simulink model "New_MPCI_JointSpace"  (R2023b)
settings: Solver=ode8  StartTime=0.0  StopTime=2  FixedStep=0.001  MaxStep=0.001  RelTol=1e-3
StopFcn:
  | clc
  | close all
  | plot(out.x_mpc,out.y_mpc,'LineWidth',1.5,'LineStyle','-.','Color','R')
  | hold on
  | plot(out.x_pid,out.y_pid,'LineWidth',1.5,'Color','B')
  | plot(out.x_d,out.y_d,'LineWidth',1.5,'LineStyle','--','Color','k')
  | legend('MPC','PID','Desired','Interpreter','tex','FontSize',15)
  | ax = gca;
  | xticklabels([-1.5 -1 -0.5 0 0.5 1 1.5 2 2.5])
  | yticklabels([141 141.5 142 142.5 143 143.5 144])
  | ax.XAxis.FontSize = 14;
  | ax.XAxis.FontWeight = 'bold';
  | ax = gca;
  | ax.YAxis.FontSize = 14;
  | ax.YAxis.FontWeight = 'bold';
  | xlabel('x(mm)','Interpreter','tex','FontSize',18,'FontWeight','bold');
  | ylabel('y(mm)','Interpreter','tex','FontSize',18,'FontWeight','bold');
  | title('End Effector Position','Interpreter','tex','FontSize',25,'FontWeight','bold');
  | grid on
  | hold off
libraries: slpidlib x1
(part 1 of 2)
settings Model: Creator=sinar  LastModifiedBy=sinar
settings SolverCC: InitialStep=0.001  ZeroCrossControl=DisableAll
settings DebuggingCC: UnconnectedInputMsg=warning  UnconnectedOutputMsg=warning  UnconnectedLineMsg=warning
settings ModelReferenceCC: EnableRefExpFcnMdlSchedulingChecks=on  ModelReferenceMinAlgLoopOccurrences=on
settings RTWCC: DLArmComputeVersion=19.05

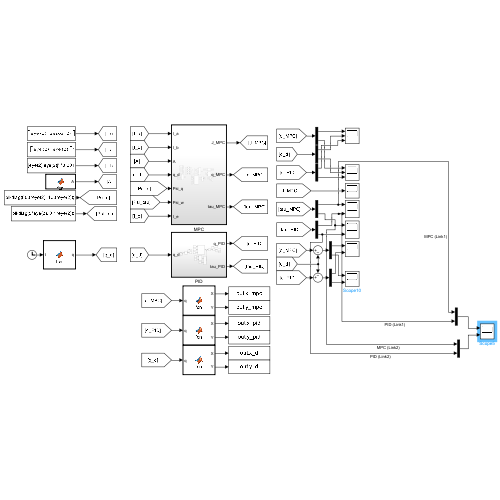
[thumbnail: Simulink's stored preview of the top-level diagram]
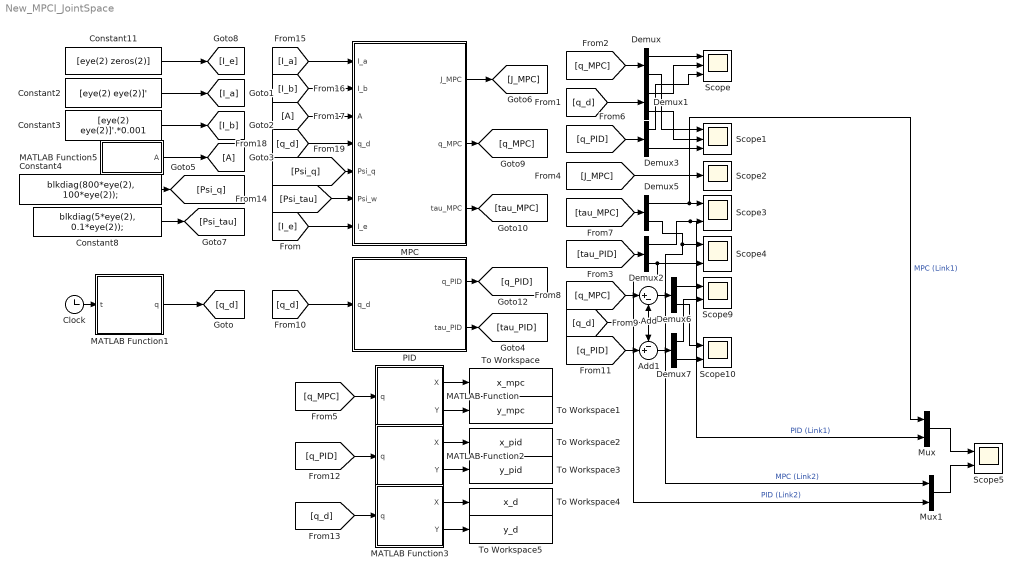
== system New_MPCI_JointSpace ==
  Add : Sum  Inputs=|+-
  Add1 : Sum  Inputs=-+|
  Clock : Clock
  Constant11 : Constant  Value=[eye(2) zeros(2)]
  Constant2 : Constant  Value=[eye(2) eye(2)]'
  Constant3 : Constant  Value=[eye(2) eye(2)]'.*0.001
  Constant4 : Constant  Value=blkdiag(800*eye(2), 100*eye(2));
  Constant8 : Constant  Value=blkdiag(5*eye(2), 0.1*eye(2));
  Demux{,1..3,5..7} (7 alike) : Demux  Outputs=2
  From17 : From
  Goto3 : Goto
  MATLAB Function : MATLAB Function  TreatAsAtomicUnit=on
  MATLAB Function1 : MATLAB Function  TreatAsAtomicUnit=on
  MATLAB Function2 : MATLAB Function  TreatAsAtomicUnit=on
  MATLAB Function3 : MATLAB Function  TreatAsAtomicUnit=on
  MATLAB Function5 : MATLAB Function  TreatAsAtomicUnit=on
  MPC : Subsystem  TreatAsAtomicUnit=on
      settings: MinAlgLoopOccurrences=on
  Mux : Mux  Inputs=2
  Mux1 : Mux  Inputs=2
  PID : Subsystem  TreatAsAtomicUnit=on
      settings: MinAlgLoopOccurrences=on
  Scope : Scope  NumInputPorts=3
  Scope1 : Scope  NumInputPorts=3
  Scope{3..5,9..10} (5 alike) : Scope  NumInputPorts=2
  Scope2 : Scope
  To Workspace : ToWorkspace  VariableName=x_mpc  SampleTime=-1
      settings: Save2DSignal=2-D array (concatenate along first dimension)
  To Workspace1 : ToWorkspace  VariableName=y_mpc  SampleTime=-1
      settings: Save2DSignal=2-D array (concatenate along first dimension)
  To Workspace2 : ToWorkspace  VariableName=x_pid  SampleTime=-1
      settings: Save2DSignal=2-D array (concatenate along first dimension)
  To Workspace3 : ToWorkspace  VariableName=y_pid  SampleTime=-1
      settings: Save2DSignal=2-D array (concatenate along first dimension)
  To Workspace4 : ToWorkspace  VariableName=x_d  SampleTime=-1
      settings: Save2DSignal=2-D array (concatenate along first dimension)
  To Workspace5 : ToWorkspace  VariableName=y_d  SampleTime=-1
      settings: Save2DSignal=2-D array (concatenate along first dimension)
  wires:
  MATLAB Function1/1(q) -> [q_d]
  Constant2/1 -> [I_a]
  Constant3/1 -> [I_b]
  MATLAB Function5/1(A) -> Goto3/1
  Constant4/1 -> [Psi_q]
  Constant8/1 -> [Psi_tau]
  Constant11/1 -> [I_e]
  MPC/1(J_MPC) -> [J_MPC]
  MPC/2(q_MPC) -> [q_MPC]
  MPC/3(tau_MPC) -> [tau_MPC]
  [Psi_tau] -> MPC/6(Psi_w)
  [Psi_q] -> MPC/5(Psi_q)
  [q_d] -> MPC/4(q_d)
  From17/1 -> MPC/3(A)
  [I_b] -> MPC/2(I_b)
  [I_a] -> MPC/1(I_a)
  Clock/1 -> MATLAB Function1/1(t)
  [I_e] -> MPC/7(I_e)
  Demux/1 -> Scope/1
  [q_d] -> Demux1/1
  [q_MPC] -> Demux/1
  [J_MPC] -> Scope2/1
  [tau_PID] -> Demux2/1
  [q_d] -> PID/1(q_d)
  PID/1(q_PID) -> [q_PID]
  PID/2(tau_PID) -> [tau_PID]
  [q_PID] -> Demux3/1
  [q_MPC] -> Add/1
  [q_d] -> Add/2, Add1/1
  [q_PID] -> Add1/2
  Add/1 -> Demux6/1
  Add1/1 -> Demux7/1
  Demux6/1 -> Scope9/1
  Demux7/1 -> Scope9/2
  Demux7/2 -> Scope10/2
  Demux6/2 -> Scope10/1
  [tau_MPC] -> Demux5/1
  Demux1/1 -> Scope/2
  Demux3/1 -> Scope/3
  Demux3/2 -> Scope1/3
  Demux1/2 -> Scope1/2
  Demux/2 -> Scope1/1
  MATLAB Function/1(X) -> To Workspace/1
  MATLAB Function/2(Y) -> To Workspace1/1
  [q_MPC] -> MATLAB Function/1(q)
  [q_PID] -> MATLAB Function2/1(q)
  MATLAB Function2/2(Y) -> To Workspace3/1
  MATLAB Function2/1(X) -> To Workspace2/1
  MATLAB Function3/1(X) -> To Workspace4/1
  MATLAB Function3/2(Y) -> To Workspace5/1
  [q_d] -> MATLAB Function3/1(q)
  Mux/1 -> Scope5/1
  Mux1/1 -> Scope5/2
  Demux2/2 -> Scope4/2, Mux1/2  "PID (Link2)"
  Demux5/2 -> Mux1/1, Scope4/1  "MPC (Link2)"
  Demux5/1 -> Mux/1, Scope3/1  "MPC (Link1)"
  Demux2/1 -> Mux/2, Scope3/2  "PID (Link1)"

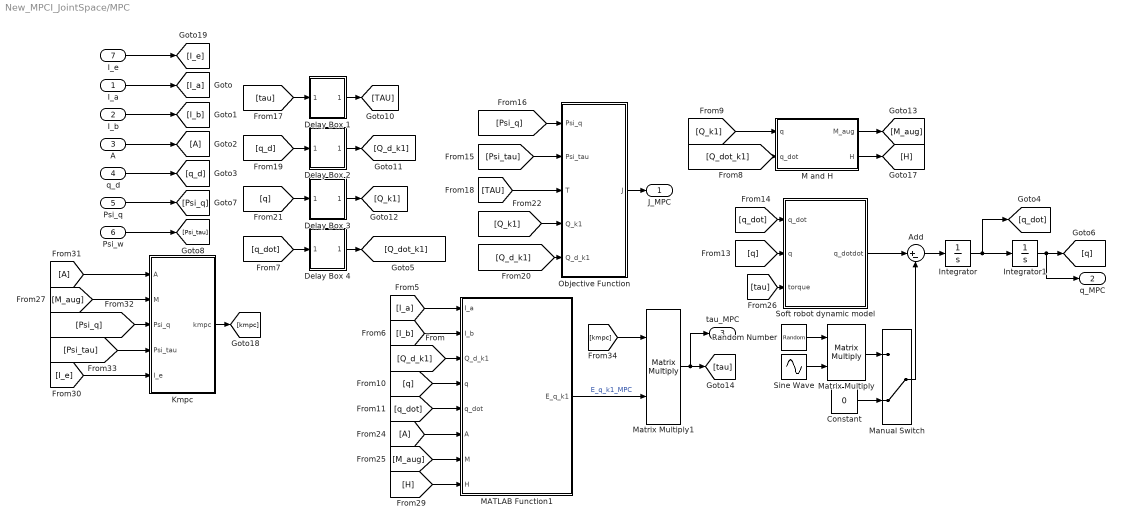
== system New_MPCI_JointSpace/MPC ==
  I_a : Inport
  I_b : Inport  Port=2
  A : Inport  Port=3
  q_d : Inport  Port=4
  Psi_q : Inport  Port=5
  Psi_w : Inport  Port=6
  I_e : Inport  Port=7
  Add : Sum  Inputs=|+-
  Constant : Constant  Value=0
  Delay Box 1 : Subsystem
  Delay Box 2 : Subsystem
  Delay Box 3 : Subsystem
  Delay Box 4 : Subsystem
  From24 : From
  From31 : From
  Goto2 : Goto
  Integrator : Integrator  InitialCondition=zeros(2,1)
  Integrator1 : Integrator  InitialCondition=[0.1 0.1]'
  Kmpc : MATLAB Function  TreatAsAtomicUnit=on
  M and H : MATLAB Function  TreatAsAtomicUnit=on
  MATLAB Function1 : MATLAB Function  TreatAsAtomicUnit=on
  Manual Switch : ManualSwitch  CurrentSetting=0
  Matrix Multiply : Product  Multiplication=Matrix(*)
  Matrix Multiply1 : Product  Multiplication=Matrix(*)
  Objective Function : MATLAB Function  TreatAsAtomicUnit=on
  Random Number : RandomNumber  Variance=5  SampleTime=0.01
  Sine Wave : Sin  Amplitude=10  Frequency=10  SampleTime=0
  Soft robot dynamic model : MATLAB Function  TreatAsAtomicUnit=on
  J_MPC : Outport
  q_MPC : Outport  Port=2
  tau_MPC : Outport  Port=3
  wires:
  Psi_q/1 -> [Psi_q]
  Psi_w/1 -> [Psi_tau]
  A/1 -> Goto2/1
  I_b/1 -> [I_b]
  I_a/1 -> [I_a]
  MATLAB Function1/1(E_q_k1) -> Matrix Multiply1/2  "E_q_k1_MPC"
  [Q_d_k1] -> Objective Function/5(Q_d_k1)
  [Q_k1] -> Objective Function/4(Q_k1)
  [tau] -> Soft robot dynamic model/3(torque)
  [Psi_tau] -> Objective Function/2(Psi_tau)
  [I_b] -> MATLAB Function1/2(I_b)
  Objective Function/1(J) -> J_MPC/1
  [Psi_q] -> Objective Function/1(Psi_q)
  Matrix Multiply1/1 -> [tau], tau_MPC/1
  [q_dot] -> Soft robot dynamic model/1(q_dot)
  Integrator1/1 -> [q], q_MPC/1
  [q_dot] -> MATLAB Function1/5(q_dot)
  [q] -> MATLAB Function1/4(q)
  [I_a] -> MATLAB Function1/1(I_a)
  Delay Box 2/1(Out1) -> [Q_d_k1]
  Delay Box 3/1(Out1) -> [Q_k1]
  [q] -> Delay Box 3/1(In1)
  Delay Box 1/1(Out1) -> [TAU]
  [tau] -> Delay Box 1/1(In1)
  Integrator/1 -> Integrator1/1, [q_dot]
  [q] -> Soft robot dynamic model/2(q)
  [q_d] -> Delay Box 2/1(In1)
  q_d/1 -> [q_d]
  [TAU] -> Objective Function/3(T)
  [q_dot] -> Delay Box 4/1(In1)
  Delay Box 4/1(Out1) -> [Q_dot_k1]
  [Q_dot_k1] -> M and H/2(q_dot)
  [Q_k1] -> M and H/1(q)
  M and H/1(M_aug) -> [M_aug]
  M and H/2(H) -> [H]
  From24/1 -> MATLAB Function1/6(A)
  [M_aug] -> MATLAB Function1/7(M)
  [H] -> MATLAB Function1/8(H)
  Kmpc/1(kmpc) -> [kmpc]
  From31/1 -> Kmpc/1(A)
  [I_e] -> Kmpc/5(I_e)
  [M_aug] -> Kmpc/2(M)
  [Psi_q] -> Kmpc/3(Psi_q)
  [kmpc] -> Matrix Multiply1/1
  I_e/1 -> [I_e]
  [Psi_tau] -> Kmpc/4(Psi_tau)
  [Q_d_k1] -> MATLAB Function1/3(Q_d_k1)
  Random Number/1 -> Matrix Multiply/1
  Sine Wave/1 -> Matrix Multiply/2
  Add/1 -> Integrator/1
  Soft robot dynamic model/1(q_dotdot) -> Add/1
  Manual Switch/1 -> Add/2
  Matrix Multiply/1 -> Manual Switch/1
  Constant/1 -> Manual Switch/2

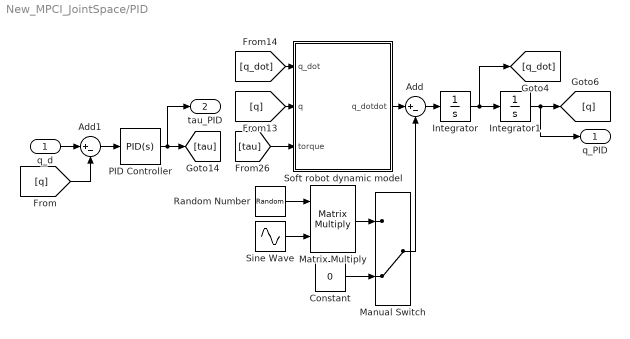
== system New_MPCI_JointSpace/PID ==
  q_d : Inport
  Add : Sum  Inputs=|+-
  Add1 : Sum  Inputs=|+-
  Constant : Constant  Value=0
  Integrator : Integrator  InitialCondition=zeros(2,1)
  Integrator1 : Integrator  InitialCondition=[0.1 0.1]'
  Manual Switch : ManualSwitch  CurrentSetting=0
  Matrix Multiply : Product  Multiplication=Matrix(*)
  PID Controller : slpidlib/PID Controller  Controller=PID  Form=Parallel  TimeDomain=Continuous-time  UseExternalTs=off  SampleTime=-1  IntegratorMethod=Forward Euler  FilterMethod=Forward Euler  ControllerParametersSource=internal  P=4  I=1  UseKiTs=off  D=0  N=100  UseFilter=on  TunerSelectOption=Transfer Function Based (PID Tuner App)  InitialConditionSource=internal  InitialConditionForIntegrator=0  InitialConditionForFilter=0  DifferentiatorICPrevScaledInput=0  ExternalReset=none  TrackingMode=off  Kt=1  LimitOutput=off  SatLimitsSource=internal  UpperSaturationLimit=inf  LowerSaturationLimit=-inf  LinearizeAsGain=on  AntiWindupMode=none  Kb=1  LimitIntegrator=off  UpperIntegratorSaturationLimit=inf  LowerIntegratorSaturationLimit=-inf  POutMin=[]  POutMax=[]  IOutMin=[]  IOutMax=[]  DOutMin=[]  DOutMax=[]  NOutMin=[]  NOutMax=[]  SumOutMin=[]  SumOutMax=[]  SaturationOutMin=[]  SaturationOutMax=[]  PParamMin=[]  PParamMax=[]  IParamMin=[]  IParamMax=[]  DParamMin=[]  DParamMax=[]  NParamMin=[]  NParamMax=[]  KbParamMin=[]  KbParamMax=[]  KtParamMin=[]  KtParamMax=[]  KbOutMin=[]  KbOutMax=[]  KtOutMin=[]  KtOutMax=[]  IntegratorOutMin=[]  IntegratorOutMax=[]  FilterOutMin=[]  FilterOutMax=[]  SumI1OutMin=[]  SumI1OutMax=[]  SumI2OutMin=[]  SumI2OutMax=[]  SumI3OutMin=[]  SumI3OutMax=[]  SumI4OutMin=[]  SumI4OutMax=[]  SumDOutMin=[]  SumDOutMax=[]  DifferentiatorOutMin=[]  DifferentiatorOutMax=[]  FilterDiffOutCoefMin=[]  FilterDiffOutCoefMax=[]  ReciprocalOutMin=[]  ReciprocalOutMax=[]  SumDenOutMin=[]  SumDenOutMax=[]  SumNumOutMin=[]  SumNumOutMax=[]  DivideOutMin=[]  DivideOutMax=[]  UdiffTsProdOutMin=[]  UdiffTsProdOutMax=[]  NTsProdOutMin=[]  NTsProdOutMax=[]  UintegralTsProdOutMin=[]  UintegralTsProdOutMax=[]  UngainTsProdOutMin=[]  UngainTsProdOutMax=[]  ClampingZeroOutDataTypeStr=Inherit: Inherit via back propagation  ClampingZeroOutMin=[]  ClampingZeroOutMax=[]  FilterDenConstantOutDataTypeStr=Inherit: Inherit via back propagation  FilterDenConstantOutMin=[]  FilterDenConstantOutMax=[]  PCopyOutDataTypeStr=Inherit: Inherit via back propagation  PCopyOutMin=[]  PCopyOutMax=[]  NCopyOutDataTypeStr=Inherit: Inherit via back propagation  NCopyOutMin=[]  NCopyOutMax=[]  IntegratorContinuousStateAttributes=''  IntegratorStateMustResolveToSignalObject=off  IntegratorRTWStateStorageClass=Auto  FilterContinuousStateAttributes=''  FilterStateMustResolveToSignalObject=off  FilterRTWStateStorageClass=Auto  ParallelPVariant=InternalParameters  IdealPVariant=Disabled  IVariant=InternalParameters  DVariant=InternalParameters  IntegratorVariant=Continuous  SatVariant=Disabled  AWVariant=Passthrough  PCopyVariant=Disabled  TRVariant=Disabled  FdbkBlocksVariant=Forward  IdealPFdbkVariant=Disabled  SatFdbkVariant=Disabled  DerivativeFilterVariant=ContFilter  NVariant=InternalParameters  NCopyVariant=Disabled  FilterICVariant=InternalICsFilter  IntegratorICVariant=InternalICs  ExternalResetVariant=Disabled  TRSumVariant=Passthrough  SumFdbkVariant=Disabled  SumVariant=Sum_PID  TsampFilterVariant=InternalTs  TsampNgainVariant=Passthrough  TsampIntegralVariant=Disabled_SignalSpec  ExternalSaturationOutDataTypeStr=Inherit: Same as second input
  Random Number : RandomNumber  Variance=5  SampleTime=0.01
  Sine Wave : Sin  Amplitude=10  Frequency=10  SampleTime=0
  Soft robot dynamic model : MATLAB Function  TreatAsAtomicUnit=on
  q_PID : Outport
  tau_PID : Outport  Port=2
  wires:
  Soft robot dynamic model/1(q_dotdot) -> Add/1
  Add/1 -> Integrator/1
  [q] -> Soft robot dynamic model/2(q)
  Integrator/1 -> Integrator1/1, [q_dot]
  Integrator1/1 -> q_PID/1, [q]
  [q_dot] -> Soft robot dynamic model/1(q_dot)
  PID Controller/1 -> tau_PID/1, [tau]
  [tau] -> Soft robot dynamic model/3(torque)
  Add1/1 -> PID Controller/1
  [q] -> Add1/2
  Random Number/1 -> Matrix Multiply/1
  Constant/1 -> Manual Switch/2
  Matrix Multiply/1 -> Manual Switch/1
  Manual Switch/1 -> Add/2
  Sine Wave/1 -> Matrix Multiply/2
  q_d/1 -> Add1/1

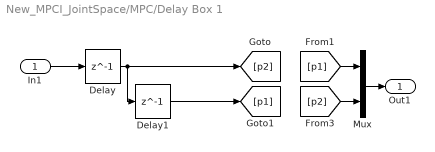
== system New_MPCI_JointSpace/MPC/Delay Box 1 ==
  In1 : Inport
  Delay : Delay  DelayLength=1  InitialCondition=[0;0]
  Delay1 : Delay  DelayLength=1  InitialCondition=[0;0]
  Mux : Mux  Inputs=2
  Out1 : Outport
  wires:
  In1/1 -> Delay/1
  [p1] -> Mux/1
  Mux/1 -> Out1/1
  [p2] -> Mux/2
  Delay1/1 -> [p1]
  Delay/1 -> Delay1/1, [p2]

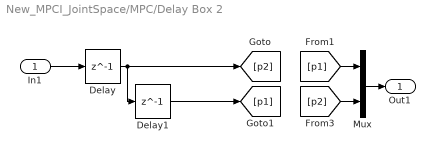
== system New_MPCI_JointSpace/MPC/Delay Box 2 ==
  In1 : Inport
  Delay : Delay  DelayLength=1  InitialCondition=[0.1;0.1];
  Delay1 : Delay  DelayLength=1  InitialCondition=[0.1;0.1];
  Mux : Mux  Inputs=2
  Out1 : Outport
  wires:
  Delay/1 -> [p2], Delay1/1
  Delay1/1 -> [p1]
  [p2] -> Mux/2
  Mux/1 -> Out1/1
  [p1] -> Mux/1
  In1/1 -> Delay/1

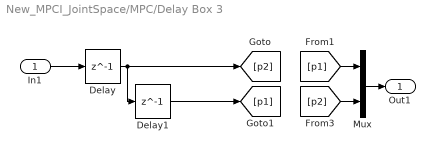
== system New_MPCI_JointSpace/MPC/Delay Box 3 ==
  In1 : Inport
  Delay : Delay  DelayLength=1  InitialCondition=[0.1;0.1];
  Delay1 : Delay  DelayLength=1  InitialCondition=[0.1;0.1];
  Mux : Mux  Inputs=2
  Out1 : Outport
  wires:
  In1/1 -> Delay/1
  [p1] -> Mux/1
  Mux/1 -> Out1/1
  [p2] -> Mux/2
  Delay1/1 -> [p1]
  Delay/1 -> Delay1/1, [p2]

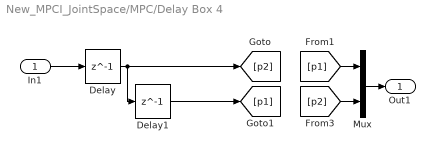
== system New_MPCI_JointSpace/MPC/Delay Box 4 ==
  In1 : Inport
  Delay : Delay  DelayLength=1  InitialCondition=[0;0]
  Delay1 : Delay  DelayLength=1  InitialCondition=[0;0]
  Mux : Mux  Inputs=2
  Out1 : Outport
  wires:
  Delay/1 -> [p2], Delay1/1
  Delay1/1 -> [p1]
  [p2] -> Mux/2
  Mux/1 -> Out1/1
  [p1] -> Mux/1
  In1/1 -> Delay/1

== matlab function New_MPCI_JointSpace/MPC/MATLAB Function1 ==
  data: I_a input; I_b input; Q_d_k1 input; E_q_k1 output; q input; q_dot input; A input; M input; H input
function E_q_k1 = fcn(I_a, I_b, Q_d_k1, q, q_dot, A, M, H)
E_q_k1 = Q_d_k1 + A*M*H - I_a*q - I_b*q_dot;

== matlab function New_MPCI_JointSpace/MPC/Objective Function ==
  data: Psi_q input; J output; Psi_tau input; T input; Q_k1 input; Q_d_k1 input
function J = fcn(Psi_q, Psi_tau, T, Q_k1, Q_d_k1)
J = transpose(Psi_q*(Q_k1-Q_d_k1))*(Psi_q*(Q_k1-Q_d_k1)) + transpose(Psi_tau*T)*(Psi_tau*T);

== matlab function New_MPCI_JointSpace/MATLAB Function1 ==
  data: t input; q output
function q  = fcn(t)
dummy = zeros(2,1);
% dummy(1) = (20*pi/180) + 0.1;
% dummy(2) = (30*pi/180) + 0.1;
% dummy(1) = (20*pi/180)*tanh(t) + 0.1;
% dummy(2) = (30*pi/180)*tanh(t) + 0.1;
% dummy(1) = (20*pi/180)*tanh(20*t) + 0.1;
% dummy(2) = (20*pi/180)*tanh(30*t) + 0.1;
% dummy(1) = (20*pi/180)/(1+exp(-0.1*t));
% dummy(2) = (30*pi/180)/(1+exp(-0.1*t));
% dummy(1) = (5*pi/180)*sin(0.1*t) + 0.1;
% dummy(2) = (10*pi/180)*sin(0.1*t) + 0.1;
if t <= 0.5
    dummy(1) = 0.1;
    dummy(2) = 0.1;
elseif  t > 0.5 && t <=1.5
    dummy(1) = 0.25*(t-0.5)+0.1;
    dummy(2) = 0.35*(t-0.5)+0.1;
else
    dummy(1) = 0.35;
    dummy(2) = 0.45;
end
q = dummy;

== matlab function New_MPCI_JointSpace/MPC/M and H ==
  data: q input; M_aug output; q_dot input; H output
function [M_aug, H] = fcn(q,q_dot)
m = 2;
mu1 = 0.02/3;
mu2 = 0.02/3;
mu3 = 0;
mu4 = 0.02/3;
l1 = 0.067;
l2 = 0.077;
mu5 = 0.0251/3;
mu6 = 0.0251/3;
mu7 = 0;
mu8 = 0.0251/3;
dummy = zeros(2*m,2*m);
dummy1 = zeros(2*m,1);
for i=1:m
    q1 = q(i+1);
    q2 = q(i+1);
    qdot1 = q_dot(i);
    qdot2 = q_dot(i+1);
    M=[ (0.25*(2.0*l1^2*mu2*q2^2 + 8.0*l1^2*mu4*q2^2 + 8.0*l1^2*mu5*q2^2 + 8.0*l1^2*mu6*q2^2 + 8.0*l1^2*mu8*q2^2 + 2.0*l2^2*mu6*q1^4 + 8.0*l2^2*mu8*q1^4 + l1^2*mu2*q1^2*q2^2 + 4.0*l1^2*mu4*q1^2*q2^2 + 4.0*l1^2*mu5*q1^2*q2^2 + 4.0*l1^2*mu6*q1^2*q2^2 + 4.0*l1^2*mu8*q1^2*q2^2 - 2.0*l1^2*mu2*q2^2*cos(q1) - 8.0*l1^2*mu4*q2^2*cos(q1) - 8.0*l1^2*mu5*q2^2*cos(q1) - 8.0*l1^2*mu6*q2^2*cos(q1) - 8.0*l1^2*mu8*q2^2*cos(q1) - 2.0*l2^2*mu6*q1^4*cos(q2) - 8.0*l2^2*mu8*q1^4*cos(q2) - 2.0*l1^2*mu2*q1*q2^2*sin(q1) - 8.0*l1^2*mu4*q1*q2^2*sin(q1) - 8.0*l1^2*mu5*q1*q2^2*sin(q1) - 8.0*l1^2*mu6*q1*q2^2*sin(q1) - 8.0*l1^2*mu8*q1*q2^2*sin(q1) - 4.0*l1*l2*mu6*q1^3*q2 - 8.0*l1*l2*mu8*q1^3*q2 - 4.0*l1*l2*mu6*q1^2*q2*sin(q1 + q2) - 8.0*l1*l2*mu8*q1^2*q2*sin(q1 + q2) + 4.0*l1*l2*mu6*q1^3*q2*cos(q2) + 8.0*l1*l2*mu8*q1^3*q2*cos(q2) + 4.0*l1*l2*mu6*q1^2*q2*sin(q1) + 4.0*l1*l2*mu6*q1^2*q2*sin(q2) + 8.0*l1*l2*mu8*q1^2*q2*sin(q1) + 8.0*l1*l2*mu8*q1^2*q2*sin(q2)))/(q1^4*q2^2), -(0.25*l2*(2.0*l1*mu6 + 4.0*l1*mu8 - 1.0*l2*mu6*q1^2 - 4.0*l2*mu8*q1^2 - 2.0*l1*mu6*cos(q1) - 2.0*l1*mu6*cos(q2) - 4.0*l1*mu8*cos(q1) - 4.0*l1*mu8*cos(q2) + 2.0*l1*mu6*cos(q1 + q2) + 4.0*l1*mu8*cos(q1 + q2) + 2.0*l1*mu6*q2*sin(q1 + q2) + 4.0*l1*mu8*q2*sin(q1 + q2) + 2.0*l1*mu6*q1*sin(q2) - 2.0*l1*mu6*q2*sin(q2) + 4.0*l1*mu8*q1*sin(q2) - 4.0*l1*mu8*q2*sin(q2) + l2*mu6*q1^2*cos(q2) + 4.0*l2*mu8*q1^2*cos(q2) - 2.0*l1*mu6*q1*q2*cos(q2) - 4.0*l1*mu8*q1*q2*cos(q2)))/(q1^2*q2^2)
                                                                                                                                                                                                                                                                                                                                                                                                                                                                                     -(0.25*l2*(2.0*l1*mu6 + 4.0*l1*mu8 - 1.0*l2*mu6*q1^2 - 4.0*l2*mu8*q1^2 - 2.0*l1*mu6*cos(q1) - 2.0*l1*mu6*cos(q2) - 4.0*l1*mu8*cos(q1) - 4.0*l1*mu8*cos(q2) + 2.0*l1*mu6*cos(q1 + q2) + 4.0*l1*mu8*cos(q1 + q2) + 2.0*l1*mu6*q2*sin(q1 + q2) + 4.0*l1*mu8*q2*sin(q1 + q2) + 2.0*l1*mu6*q1*sin(q2) - 2.0*l1*mu6*q2*sin(q2) + 4.0*l1*mu8*q1*sin(q2) - 4.0*l1*mu8*q2*sin(q2) + l2*mu6*q1^2*cos(q2) + 4.0*l2*mu8*q1^2*cos(q2) - 2.0*l1*mu6*q1*q2*cos(q2) - 4.0*l1*mu8*q1*q2*cos(q2)))/(q1^2*q2^2),                                                                                                                                                                                                                                                                                                                                                                                                            -(0.25*l2^2*(mu6 + 4.0*mu8)*(2.0*cos(q2) + 2.0*q2*sin(q2) - 1.0*q2^2 - 2.0))/q2^4];
    C_q=[-(0.5*(2.0*l1^2*mu2*q2^3*qdot1^2 + 8.0*l1^2*mu4*q2^3*qdot1^2 + 8.0*l1^2*mu5*q2^3*qdot1^2 + 8.0*l1^2*mu6*q2^3*qdot1^2 + 8.0*l1^2*mu8*q2^3*qdot1^2 + l2^2*mu6*q1^5*qdot2^2 + 4.0*l2^2*mu8*q1^5*qdot2^2 + 0.5*l1^2*mu2*q1^2*q2^3*qdot1^2 + 2.0*l1^2*mu4*q1^2*q2^3*qdot1^2 + 2.0*l1^2*mu5*q1^2*q2^3*qdot1^2 + 2.0*l1^2*mu6*q1^2*q2^3*qdot1^2 + 2.0*l1^2*mu8*q1^2*q2^3*qdot1^2 - 2.0*l1^2*mu2*q2^3*qdot1^2*cos(q1) - 8.0*l1^2*mu4*q2^3*qdot1^2*cos(q1) - 8.0*l1^2*mu5*q2^3*qdot1^2*cos(q1) - 8.0*l1^2*mu6*q2^3*qdot1^2*cos(q1) - 8.0*l1^2*mu8*q2^3*qdot1^2*cos(q1) - 1.0*l2^2*mu6*q1^5*qdot2^2*cos(q2) - 4.0*l2^2*mu8*q1^5*qdot2^2*cos(q2) - 2.0*l1*l2*mu6*q1^3*qdot2^2 - 4.0*l1*l2*mu8*q1^3*qdot2^2 + 2.0*l2^2*mu6*q1^5*qdot1*qdot2 + 8.0*l2^2*mu8*q1^5*qdot1*qdot2 - 1.0*l1*l2*mu6*q1^3*q2^2*qdot1^2 - 2.0*l1*l2*mu8*q1^3*q2^2*qdot1^2 + 2.0*l1*l2*mu6*q1^3*qdot2^2*cos(q1) + 2.0*l1*l2*mu6*q1^3*qdot2^2*cos(q2) + 4.0*l1*l2*mu8*q1^3*qdot2^2*cos(q1) + 4.0*l1*l2*mu8*q1^3*qdot2^2*cos(q2) - 2.0*l2^2*mu6*q1^5*qdot1*qdot2*cos(q2) - 8.0*l2^2*mu8*q1^5*qdot1*qdot2*cos(q2) - 2.0*l1*l2*mu6*q1^4*qdot2^2*sin(q2) - 4.0*l1*l2*mu8*q1^4*qdot2^2*sin(q2) - 2.0*l1^2*mu2*q1*q2^3*qdot1^2*sin(q1) - 8.0*l1^2*mu4*q1*q2^3*qdot1^2*sin(q1) - 8.0*l1^2*mu5*q1*q2^3*qdot1^2*sin(q1) - 8.0*l1^2*mu6*q1*q2^3*qdot1^2*sin(q1) - 8.0*l1^2*mu8*q1*q2^3*qdot1^2*sin(q1) - 0.5*l2^2*mu6*q1^5*q2*qdot2^2*sin(q2) - 2.0*l2^2*mu8*q1^5*q2*qdot2^2*sin(q2) + 0.5*l1^2*mu2*q1^2*q2^3*qdot1^2*cos(q1) + 2.0*l1^2*mu4*q1^2*q2^3*qdot1^2*cos(q1) + 2.0*l1^2*mu5*q1^2*q2^3*qdot1^2*cos(q1) + 2.0*l1^2*mu6*q1^2*q2^3*qdot1^2*cos(q1) + 2.0*l1^2*mu8*q1^2*q2^3*qdot1^2*cos(q1) - 2.0*l1*l2*mu6*q1^3*qdot2^2*cos(q1 + q2) - 4.0*l1*l2*mu8*q1^3*qdot2^2*cos(q1 + q2) - 2.0*l1*l2*mu6*q1^3*q2*qdot2^2*sin(q1 + q2) - 4.0*l1*l2*mu8*q1^3*q2*qdot2^2*sin(q1 + q2) + 2.0*l1*l2*mu6*q1^4*q2*qdot2^2*cos(q2) + 4.0*l1*l2*mu8*q1^4*q2*qdot2^2*cos(q2) + 2.0*l1*l2*mu6*q1^3*q2*qdot2^2*sin(q2) + 4.0*l1*l2*mu8*q1^3*q2*qdot2^2*sin(q2) - 1.0*l2^2*mu6*q1^5*q2*qdot1*qdot2*sin(q2) - 4.0*l2^2*mu8*q1^5*q2*qdot1*qdot2*sin(q2) + l1*l2*mu6*q1^3*q2^2*qdot1^2*cos(q1 + q2) + l1*l2*mu6*q1^3*q2^2*qdot2^2*cos(q1 + q2) + 2.0*l1*l2*mu8*q1^3*q2^2*qdot1^2*cos(q1 + q2) + 2.0*l1*l2*mu8*q1^3*q2^2*qdot2^2*cos(q1 + q2) - 2.0*l1*l2*mu6*q1^4*q2*qdot1*qdot2 - 4.0*l1*l2*mu8*q1^4*q2*qdot1*qdot2 - 2.0*l1*l2*mu6*q1^2*q2^2*qdot1^2*sin(q1 + q2) - 4.0*l1*l2*mu8*q1^2*q2^2*qdot1^2*sin(q1 + q2) - 1.0*l1*l2*mu6*q1^3*q2^2*qdot1^2*cos(q1) + l1*l2*mu6*q1^3*q2^2*qdot1^2*cos(q2) - 1.0*l1*l2*mu6*q1^3*q2^2*qdot2^2*cos(q2) - 2.0*l1*l2*mu8*q1^3*q2^2*qdot1^2*cos(q1) + 2.0*l1*l2*mu8*q1^3*q2^2*qdot1^2*cos(q2) - 2.0*l1*l2*mu8*q1^3*q2^2*qdot2^2*cos(q2) + 2.0*l1*l2*mu6*q1^2*q2^2*qdot1^2*sin(q1) + 2.0*l1*l2*mu6*q1^2*q2^2*qdot1^2*sin(q2) + 4.0*l1*l2*mu8*q1^2*q2^2*qdot1^2*sin(q1) + 4.0*l1*l2*mu8*q1^2*q2^2*qdot1^2*sin(q2) + l1*l2*mu6*q1^4*q2^2*qdot2^2*sin(q2) + 2.0*l1*l2*mu8*q1^4*q2^2*qdot2^2*sin(q2) + 2.0*l1*l2*mu6*q1^4*q2^2*qdot1*qdot2*sin(q2) + 4.0*l1*l2*mu8*q1^4*q2^2*qdot1*qdot2*sin(q2) - 2.0*l1*l2*mu6*q1^3*q2*qdot1*qdot2*sin(q1 + q2) - 4.0*l1*l2*mu8*q1^3*q2*qdot1*qdot2*sin(q1 + q2) + 2.0*l1*l2*mu6*q1^4*q2*qdot1*qdot2*cos(q2) + 4.0*l1*l2*mu8*q1^4*q2*qdot1*qdot2*cos(q2) + 2.0*l1*l2*mu6*q1^3*q2*qdot1*qdot2*sin(q1) + 2.0*l1*l2*mu6*q1^3*q2*qdot1*qdot2*sin(q2) + 4.0*l1*l2*mu8*q1^3*q2*qdot1*qdot2*sin(q1) + 4.0*l1*l2*mu8*q1^3*q2*qdot1*qdot2*sin(q2) + 2.0*l1*l2*mu6*q1^3*q2^2*qdot1*qdot2*cos(q1 + q2) + 4.0*l1*l2*mu8*q1^3*q2^2*qdot1*qdot2*cos(q1 + q2) - 2.0*l1*l2*mu6*q1^3*q2^2*qdot1*qdot2*cos(q2) - 4.0*l1*l2*mu8*q1^3*q2^2*qdot1*qdot2*cos(q2)))/(q1^5*q2^3)
                                                                                                                                                                                                                                                                                                                                                                                                                                                                                                                                                                                                                                                                                                                                                                                                                                                                                                                                                                                                                                                                                                                                                                                                                                                                                                                                                                                                                                                                                                                                                                                                                                                                                                                                                                                                                                                                                                                                                                                                                                                                                                                                                                                                                                                     -(0.25*l2*(4.0*l2*mu6*q1^3*qdot2^2 - 4.0*l1*mu6*q2^3*qdot1^2 - 8.0*l1*mu8*q2^3*qdot1^2 + 16.0*l2*mu8*q1^3*qdot2^2 - 4.0*l1*mu6*q2^3*qdot1^2*cos(q1 + q2) - 8.0*l1*mu8*q2^3*qdot1^2*cos(q1 + q2) - 4.0*l1*mu6*q2^4*qdot1^2*sin(q1 + q2) - 8.0*l1*mu8*q2^4*qdot1^2*sin(q1 + q2) + 2.0*l1*mu6*q1^2*q2^3*qdot1^2 - 2.0*l2*mu6*q1^3*q2^2*qdot1^2 + 4.0*l1*mu8*q1^2*q2^3*qdot1^2 + l2*mu6*q1^3*q2^2*qdot2^2 - 8.0*l2*mu8*q1^3*q2^2*qdot1^2 + 4.0*l2*mu8*q1^3*q2^2*qdot2^2 + 4.0*l1*mu6*q2^3*qdot1^2*cos(q1) + 4.0*l1*mu6*q2^3*qdot1^2*cos(q2) + 8.0*l1*mu8*q2^3*qdot1^2*cos(q1) - 4.0*l2*mu6*q1^3*qdot2^2*cos(q2) + 8.0*l1*mu8*q2^3*qdot1^2*cos(q2) - 16.0*l2*mu8*q1^3*qdot2^2*cos(q2) + 4.0*l1*mu6*q2^4*qdot1^2*sin(q2) + 8.0*l1*mu8*q2^4*qdot1^2*sin(q2) + 4.0*l1*mu6*q1*q2^4*qdot1^2*cos(q2) + 8.0*l1*mu8*q1*q2^4*qdot1^2*cos(q2) - 4.0*l1*mu6*q1*q2^3*qdot1^2*sin(q2) - 8.0*l1*mu8*q1*q2^3*qdot1^2*sin(q2) - 4.0*l2*mu6*q1^3*q2*qdot2^2*sin(q2) - 16.0*l2*mu8*q1^3*q2*qdot2^2*sin(q2) - 2.0*l1*mu6*q1^2*q2^3*qdot1^2*cos(q2) + 2.0*l2*mu6*q1^3*q2^2*qdot1^2*cos(q2) - 4.0*l1*mu8*q1^2*q2^3*qdot1^2*cos(q2) + l2*mu6*q1^3*q2^2*qdot2^2*cos(q2) + 8.0*l2*mu8*q1^3*q2^2*qdot1^2*cos(q2) + 4.0*l2*mu8*q1^3*q2^2*qdot2^2*cos(q2) - 2.0*l1*mu6*q1^2*q2^4*qdot1^2*sin(q2) + l2*mu6*q1^3*q2^3*qdot1^2*sin(q2) - 4.0*l1*mu8*q1^2*q2^4*qdot1^2*sin(q2) + 4.0*l2*mu8*q1^3*q2^3*qdot1^2*sin(q2)))/(q1^3*q2^5)];
    G=[-(0.005*(981.0*l2*q1^2*cos(q1 + q2)*conj(mu6) + 1962.0*l2*q1^2*cos(q1 + q2)*conj(mu8) - 981.0*l2*q1^2*conj(mu6)*cos(q1) - 1962.0*l2*q1^2*conj(mu8)*cos(q1) - 981.0*l1*mu2*q2*sin(q1) - 1962.0*l1*q2*conj(mu4)*sin(q1) - 1962.0*l1*q2*conj(mu5)*sin(q1) - 1962.0*l1*q2*conj(mu6)*sin(q1) - 1962.0*l1*q2*conj(mu8)*sin(q1) + 1962.0*l1*q1*q2*conj(mu4)*cos(q1) + 1962.0*l1*q1*q2*conj(mu5)*cos(q1) + 1962.0*l1*q1*q2*conj(mu6)*cos(q1) + 1962.0*l1*q1*q2*conj(mu8)*cos(q1) + 981.0*l1*mu2*q1*q2*cos(q1)))/(q1^2*q2)
                                                                                                                                                                                                                                                                                                                                                                                                                           -(4.905*l2*(conj(mu6) + 2.0*conj(mu8))*(sin(q1) - 1.0*sin(q1 + q2) + q2*cos(q1 + q2)))/q2^2];
    K=[0.68,0;0,0.7];
    D=[0.0029,0;0,0.003];
    h = K*[q1;q2]+D*[qdot1;qdot2]+C_q+G;
    dummy(2*i-1:2*i,2*i-1:2*i) = inv(M);
    dummy1(2*i-1:2*i) =  h;
end
H = dummy1;
M_aug = dummy;

== matlab function New_MPCI_JointSpace/MATLAB Function ==
  data: q input; X output; Y output
function [X,Y] = fcn(q)
T1 = [cos(q(1)) -sin(q(1)) 0.067*(1-cos(q(1)))/q(1);
      sin(q(1)) cos(q(1)) 0.067*(sin(q(1)))/q(1);
      0 0 1];
T2 = [cos(q(2)) -sin(q(2)) 0.077*(1-cos(q(2)))/q(2);
      sin(q(2)) cos(q(2)) 0.077*(sin(q(2)))/q(2);
      0 0 1];
T = T1*T2;
X = T(1,3);
Y = T(2,3);

== matlab function New_MPCI_JointSpace/MPC/Kmpc ==
  data: A input; M input; kmpc output; Psi_q input; Psi_tau input; I_e input
function kmpc = fcn(A, M, Psi_q, Psi_tau, I_e)
P = transpose(Psi_q*A*M)*(Psi_q*A*M) + transpose(Psi_tau)*Psi_tau;
Kmpc = pinv(P)*transpose(Psi_q*A*M)*Psi_q;
kmpc = I_e * Kmpc;

== matlab function New_MPCI_JointSpace/MATLAB Function2 ==
  data: q input; X output; Y output
function [X,Y] = fcn(q)
T1 = [cos(q(1)) -sin(q(1)) 0.067*(1-cos(q(1)))/q(1);
      sin(q(1)) cos(q(1)) 0.067*(sin(q(1)))/q(1);
      0 0 1];
T2 = [cos(q(2)) -sin(q(2)) 0.077*(1-cos(q(2)))/q(2);
      sin(q(2)) cos(q(2)) 0.077*(sin(q(2)))/q(2);
      0 0 1];
T = T1*T2;
X = T(1,3);
Y = T(2,3);

== matlab function New_MPCI_JointSpace/MATLAB Function3 ==
  data: q input; X output; Y output
function [X,Y] = fcn(q)
T1 = [cos(q(1)) -sin(q(1)) 0.067*(1-cos(q(1)))/q(1);
      sin(q(1)) cos(q(1)) 0.067*(sin(q(1)))/q(1);
      0 0 1];
T2 = [cos(q(2)) -sin(q(2)) 0.077*(1-cos(q(2)))/q(2);
      sin(q(2)) cos(q(2)) 0.077*(sin(q(2)))/q(2);
      0 0 1];
T = T1*T2;
X = T(1,3);
Y = T(2,3);

== matlab function New_MPCI_JointSpace/MATLAB Function5 ==
  data: A output
function A = fcn()
% A = [0.5*eye(2) zeros(2) zeros(2);
%     1.5*eye(2) 0.5*eye(2) zeros(2);
%     2.5*eye(2) 1.5*eye(2) 0.5*eye(2)].*0.001^2;
A = [0.5*eye(2) zeros(2);
    1.5*eye(2) 0.5*eye(2)].*0.001^2;

== matlab function New_MPCI_JointSpace/MPC/Soft robot dynamic model ==
  data: q_dot input; q input; q_dotdot output; torque input
function q_dotdot  = fcn(q_dot,q,torque)

mu1 = 0.02/3;
mu2 = 0.02/3;
mu3 = 0;
mu4 = 0.02/3;
l1 = 0.067;
l2 = 0.077;
mu5 = 0.0251/3;
mu6 = 0.0251/3;
mu7 = 0;
mu8 = 0.0251/3;

q1 = q(1);
q2 = q(2);
qdot1 = q_dot(1);
qdot2 = q_dot(2);

M=[ (0.25*(2.0*l1^2*mu2*q2^2 + 8.0*l1^2*mu4*q2^2 + 8.0*l1^2*mu5*q2^2 + 8.0*l1^2*mu6*q2^2 + 8.0*l1^2*mu8*q2^2 + 2.0*l2^2*mu6*q1^4 + 8.0*l2^2*mu8*q1^4 + l1^2*mu2*q1^2*q2^2 + 4.0*l1^2*mu4*q1^2*q2^2 + 4.0*l1^2*mu5*q1^2*q2^2 + 4.0*l1^2*mu6*q1^2*q2^2 + 4.0*l1^2*mu8*q1^2*q2^2 - 2.0*l1^2*mu2*q2^2*cos(q1) - 8.0*l1^2*mu4*q2^2*cos(q1) - 8.0*l1^2*mu5*q2^2*cos(q1) - 8.0*l1^2*mu6*q2^2*cos(q1) - 8.0*l1^2*mu8*q2^2*cos(q1) - 2.0*l2^2*mu6*q1^4*cos(q2) - 8.0*l2^2*mu8*q1^4*cos(q2) - 2.0*l1^2*mu2*q1*q2^2*sin(q1) - 8.0*l1^2*mu4*q1*q2^2*sin(q1) - 8.0*l1^2*mu5*q1*q2^2*sin(q1) - 8.0*l1^2*mu6*q1*q2^2*sin(q1) - 8.0*l1^2*mu8*q1*q2^2*sin(q1) - 4.0*l1*l2*mu6*q1^3*q2 - 8.0*l1*l2*mu8*q1^3*q2 - 4.0*l1*l2*mu6*q1^2*q2*sin(q1 + q2) - 8.0*l1*l2*mu8*q1^2*q2*sin(q1 + q2) + 4.0*l1*l2*mu6*q1^3*q2*cos(q2) + 8.0*l1*l2*mu8*q1^3*q2*cos(q2) + 4.0*l1*l2*mu6*q1^2*q2*sin(q1) + 4.0*l1*l2*mu6*q1^2*q2*sin(q2) + 8.0*l1*l2*mu8*q1^2*q2*sin(q1) + 8.0*l1*l2*mu8*q1^2*q2*sin(q2)))/(q1^4*q2^2), -(0.25*l2*(2.0*l1*mu6 + 4.0*l1*mu8 - 1.0*l2*mu6*q1^2 - 4.0*l2*mu8*q1^2 - 2.0*l1*mu6*cos(q1) - 2.0*l1*mu6*cos(q2) - 4.0*l1*mu8*cos(q1) - 4.0*l1*mu8*cos(q2) + 2.0*l1*mu6*cos(q1 + q2) + 4.0*l1*mu8*cos(q1 + q2) + 2.0*l1*mu6*q2*sin(q1 + q2) + 4.0*l1*mu8*q2*sin(q1 + q2) + 2.0*l1*mu6*q1*sin(q2) - 2.0*l1*mu6*q2*sin(q2) + 4.0*l1*mu8*q1*sin(q2) - 4.0*l1*mu8*q2*sin(q2) + l2*mu6*q1^2*cos(q2) + 4.0*l2*mu8*q1^2*cos(q2) - 2.0*l1*mu6*q1*q2*cos(q2) - 4.0*l1*mu8*q1*q2*cos(q2)))/(q1^2*q2^2)
                                                                                                                                                                                                                                                                                                                                                                                                                                                                                     -(0.25*l2*(2.0*l1*mu6 + 4.0*l1*mu8 - 1.0*l2*mu6*q1^2 - 4.0*l2*mu8*q1^2 - 2.0*l1*mu6*cos(q1) - 2.0*l1*mu6*cos(q2) - 4.0*l1*mu8*cos(q1) - 4.0*l1*mu8*cos(q2) + 2.0*l1*mu6*cos(q1 + q2) + 4.0*l1*mu8*cos(q1 + q2) + 2.0*l1*mu6*q2*sin(q1 + q2) + 4.0*l1*mu8*q2*sin(q1 + q2) + 2.0*l1*mu6*q1*sin(q2) - 2.0*l1*mu6*q2*sin(q2) + 4.0*l1*mu8*q1*sin(q2) - 4.0*l1*mu8*q2*sin(q2) + l2*mu6*q1^2*cos(q2) + 4.0*l2*mu8*q1^2*cos(q2) - 2.0*l1*mu6*q1*q2*cos(q2) - 4.0*l1*mu8*q1*q2*cos(q2)))/(q1^2*q2^2),                                                                                                                                                                                                                                                                                                                                                                                                            -(0.25*l2^2*(mu6 + 4.0*mu8)*(2.0*cos(q2) + 2.0*q2*sin(q2) - 1.0*q2^2 - 2.0))/q2^4];

C_q=[-(0.5*(2.0*l1^2*mu2*q2^3*qdot1^2 + 8.0*l1^2*mu4*q2^3*qdot1^2 + 8.0*l1^2*mu5*q2^3*qdot1^2 + 8.0*l1^2*mu6*q2^3*qdot1^2 + 8.0*l1^2*mu8*q2^3*qdot1^2 + l2^2*mu6*q1^5*qdot2^2 + 4.0*l2^2*mu8*q1^5*qdot2^2 + 0.5*l1^2*mu2*q1^2*q2^3*qdot1^2 + 2.0*l1^2*mu4*q1^2*q2^3*qdot1^2 + 2.0*l1^2*mu5*q1^2*q2^3*qdot1^2 + 2.0*l1^2*mu6*q1^2*q2^3*qdot1^2 + 2.0*l1^2*mu8*q1^2*q2^3*qdot1^2 - 2.0*l1^2*mu2*q2^3*qdot1^2*cos(q1) - 8.0*l1^2*mu4*q2^3*qdot1^2*cos(q1) - 8.0*l1^2*mu5*q2^3*qdot1^2*cos(q1) - 8.0*l1^2*mu6*q2^3*qdot1^2*cos(q1) - 8.0*l1^2*mu8*q2^3*qdot1^2*cos(q1) - 1.0*l2^2*mu6*q1^5*qdot2^2*cos(q2) - 4.0*l2^2*mu8*q1^5*qdot2^2*cos(q2) - 2.0*l1*l2*mu6*q1^3*qdot2^2 - 4.0*l1*l2*mu8*q1^3*qdot2^2 + 2.0*l2^2*mu6*q1^5*qdot1*qdot2 + 8.0*l2^2*mu8*q1^5*qdot1*qdot2 - 1.0*l1*l2*mu6*q1^3*q2^2*qdot1^2 - 2.0*l1*l2*mu8*q1^3*q2^2*qdot1^2 + 2.0*l1*l2*mu6*q1^3*qdot2^2*cos(q1) + 2.0*l1*l2*mu6*q1^3*qdot2^2*cos(q2) + 4.0*l1*l2*mu8*q1^3*qdot2^2*cos(q1) + 4.0*l1*l2*mu8*q1^3*qdot2^2*cos(q2) - 2.0*l2^2*mu6*q1^5*qdot1*qdot2*cos(q2) - 8.0*l2^2*mu8*q1^5*qdot1*qdot2*cos(q2) - 2.0*l1*l2*mu6*q1^4*qdot2^2*sin(q2) - 4.0*l1*l2*mu8*q1^4*qdot2^2*sin(q2) - 2.0*l1^2*mu2*q1*q2^3*qdot1^2*sin(q1) - 8.0*l1^2*mu4*q1*q2^3*qdot1^2*sin(q1) - 8.0*l1^2*mu5*q1*q2^3*qdot1^2*sin(q1) - 8.0*l1^2*mu6*q1*q2^3*qdot1^2*sin(q1) - 8.0*l1^2*mu8*q1*q2^3*qdot1^2*sin(q1) - 0.5*l2^2*mu6*q1^5*q2*qdot2^2*sin(q2) - 2.0*l2^2*mu8*q1^5*q2*qdot2^2*sin(q2) + 0.5*l1^2*mu2*q1^2*q2^3*qdot1^2*cos(q1) + 2.0*l1^2*mu4*q1^2*q2^3*qdot1^2*cos(q1) + 2.0*l1^2*mu5*q1^2*q2^3*qdot1^2*cos(q1) + 2.0*l1^2*mu6*q1^2*q2^3*qdot1^2*cos(q1) + 2.0*l1^2*mu8*q1^2*q2^3*qdot1^2*cos(q1) - 2.0*l1*l2*mu6*q1^3*qdot2^2*cos(q1 + q2) - 4.0*l1*l2*mu8*q1^3*qdot2^2*cos(q1 + q2) - 2.0*l1*l2*mu6*q1^3*q2*qdot2^2*sin(q1 + q2) - 4.0*l1*l2*mu8*q1^3*q2*qdot2^2*sin(q1 + q2) + 2.0*l1*l2*mu6*q1^4*q2*qdot2^2*cos(q2) + 4.0*l1*l2*mu8*q1^4*q2*qdot2^2*cos(q2) + 2.0*l1*l2*mu6*q1^3*q2*qdot2^2*sin(q2) + 4.0*l1*l2*mu8*q1^3*q2*qdot2^2*sin(q2) - 1.0*l2^2*mu6*q1^5*q2*qdot1*qdot2*sin(q2) - 4.0*l2^2*mu8*q1^5*q2*qdot1*qdot2*sin(q2) + l1*l2*mu6*q1^3*q2^2*qdot1^2*cos(q1 + q2) + l1*l2*mu6*q1^3*q2^2*qdot2^2*cos(q1 + q2) + 2.0*l1*l2*mu8*q1^3*q2^2*qdot1^2*cos(q1 + q2) + 2.0*l1*l2*mu8*q1^3*q2^2*qdot2^2*cos(q1 + q2) - 2.0*l1*l2*mu6*q1^4*q2*qdot1*qdot2 - 4.0*l1*l2*mu8*q1^4*q2*qdot1*qdot2 - 2.0*l1*l2*mu6*q1^2*q2^2*qdot1^2*sin(q1 + q2) - 4.0*l1*l2*mu8*q1^2*q2^2*qdot1^2*sin(q1 + q2) - 1.0*l1*l2*mu6*q1^3*q2^2*qdot1^2*cos(q1) + l1*l2*mu6*q1^3*q2^2*qdot1^2*cos(q2) - 1.0*l1*l2*mu6*q1^3*q2^2*qdot2^2*cos(q2) - 2.0*l1*l2*mu8*q1^3*q2^2*qdot1^2*cos(q1) + 2.0*l1*l2*mu8*q1^3*q2^2*qdot1^2*cos(q2) - 2.0*l1*l2*mu8*q1^3*q2^2*qdot2^2*cos(q2) + 2.0*l1*l2*mu6*q1^2*q2^2*qdot1^2*sin(q1) + 2.0*l1*l2*mu6*q1^2*q2^2*qdot1^2*sin(q2) + 4.0*l1*l2*mu8*q1^2*q2^2*qdot1^2*sin(q1) + 4.0*l1*l2*mu8*q1^2*q2^2*qdot1^2*sin(q2) + l1*l2*mu6*q1^4*q2^2*qdot2^2*sin(q2) + 2.0*l1*l2*mu8*q1^4*q2^2*qdot2^2*sin(q2) + 2.0*l1*l2*mu6*q1^4*q2^2*qdot1*qdot2*sin(q2) + 4.0*l1*l2*mu8*q1^4*q2^2*qdot1*qdot2*sin(q2) - 2.0*l1*l2*mu6*q1^3*q2*qdot1*qdot2*sin(q1 + q2) - 4.0*l1*l2*mu8*q1^3*q2*qdot1*qdot2*sin(q1 + q2) + 2.0*l1*l2*mu6*q1^4*q2*qdot1*qdot2*cos(q2) + 4.0*l1*l2*mu8*q1^4*q2*qdot1*qdot2*cos(q2) + 2.0*l1*l2*mu6*q1^3*q2*qdot1*qdot2*sin(q1) + 2.0*l1*l2*mu6*q1^3*q2*qdot1*qdot2*sin(q2) + 4.0*l1*l2*mu8*q1^3*q2*qdot1*qdot2*sin(q1) + 4.0*l1*l2*mu8*q1^3*q2*qdot1*qdot2*sin(q2) + 2.0*l1*l2*mu6*q1^3*q2^2*qdot1*qdot2*cos(q1 + q2) + 4.0*l1*l2*mu8*q1^3*q2^2*qdot1*qdot2*cos(q1 + q2) - 2.0*l1*l2*mu6*q1^3*q2^2*qdot1*qdot2*cos(q2) - 4.0*l1*l2*mu8*q1^3*q2^2*qdot1*qdot2*cos(q2)))/(q1^5*q2^3)
                                                                                                                                                                                                                                                                                                                                                                                                                                                                                                                                                                                                                                                                                                                                                                                                                                                                                                                                                                                                                                                                                                                                                                                                                                                                                                                                                                                                                                                                                                                                                                                                                                                                                                                                                                                                                                                                                                                                                                                                                                                                                                                                                                                                                                                     -(0.25*l2*(4.0*l2*mu6*q1^3*qdot2^2 - 4.0*l1*mu6*q2^3*qdot1^2 - 8.0*l1*mu8*q2^3*qdot1^2 + 16.0*l2*mu8*q1^3*qdot2^2 - 4.0*l1*mu6*q2^3*qdot1^2*cos(q1 + q2) - 8.0*l1*mu8*q2^3*qdot1^2*cos(q1 + q2) - 4.0*l1*mu6*q2^4*qdot1^2*sin(q1 + q2) - 8.0*l1*mu8*q2^4*qdot1^2*sin(q1 + q2) + 2.0*l1*mu6*q1^2*q2^3*qdot1^2 - 2.0*l2*mu6*q1^3*q2^2*qdot1^2 + 4.0*l1*mu8*q1^2*q2^3*qdot1^2 + l2*mu6*q1^3*q2^2*qdot2^2 - 8.0*l2*mu8*q1^3*q2^2*qdot1^2 + 4.0*l2*mu8*q1^3*q2^2*qdot2^2 + 4.0*l1*mu6*q2^3*qdot1^2*cos(q1) + 4.0*l1*mu6*q2^3*qdot1^2*cos(q2) + 8.0*l1*mu8*q2^3*qdot1^2*cos(q1) - 4.0*l2*mu6*q1^3*qdot2^2*cos(q2) + 8.0*l1*mu8*q2^3*qdot1^2*cos(q2) - 16.0*l2*mu8*q1^3*qdot2^2*cos(q2) + 4.0*l1*mu6*q2^4*qdot1^2*sin(q2) + 8.0*l1*mu8*q2^4*qdot1^2*sin(q2) + 4.0*l1*mu6*q1*q2^4*qdot1^2*cos(q2) + 8.0*l1*mu8*q1*q2^4*qdot1^2*cos(q2) - 4.0*l1*mu6*q1*q2^3*qdot1^2*sin(q2) - 8.0*l1*mu8*q1*q2^3*qdot1^2*sin(q2) - 4.0*l2*mu6*q1^3*q2*qdot2^2*sin(q2) - 16.0*l2*mu8*q1^3*q2*qdot2^2*sin(q2) - 2.0*l1*mu6*q1^2*q2^3*qdot1^2*cos(q2) + 2.0*l2*mu6*q1^3*q2^2*qdot1^2*cos(q2) - 4.0*l1*mu8*q1^2*q2^3*qdot1^2*cos(q2) + l2*mu6*q1^3*q2^2*qdot2^2*cos(q2) + 8.0*l2*mu8*q1^3*q2^2*qdot1^2*cos(q2) + 4.0*l2*mu8*q1^3*q2^2*qdot2^2*cos(q2) - 2.0*l1*mu6*q1^2*q2^4*qdot1^2*sin(q2) + l2*mu6*q1^3*q2^3*qdot1^2*sin(q2) - 4.0*l1*mu8*q1^2*q2^4*qdot1^2*sin(q2) + 4.0*l2*mu8*q1^3*q2^3*qdot1^2*sin(q2)))/(q1^3*q2^5)];
                                                                                                                                                                                                                                                                                                                                                                                                                                                                                                                                                                                                                                                                                                                                                                                                                                                                                                                                                                                                                                                                                                  
G=[-(0.005*(981.0*l2*q1^2*cos(q1 + q2)*conj(mu6) + 1962.0*l2*q1^2*cos(q1 + q2)*conj(mu8) - 981.0*l2*q1^2*conj(mu6)*cos(q1) - 1962.0*l2*q1^2*conj(mu8)*cos(q1) - 981.0*l1*mu2*q2*sin(q1) - 1962.0*l1*q2*conj(mu4)*sin(q1) - 1962.0*l1*q2*conj(mu5)*sin(q1) - 1962.0*l1*q2*conj(mu6)*sin(q1) - 1962.0*l1*q2*conj(mu8)*sin(q1) + 1962.0*l1*q1*q2*conj(mu4)*cos(q1) + 1962.0*l1*q1*q2*conj(mu5)*cos(q1) + 1962.0*l1*q1*q2*conj(mu6)*cos(q1) + 1962.0*l1*q1*q2*conj(mu8)*cos(q1) + 981.0*l1*mu2*q1*q2*cos(q1)))/(q1^2*q2)
                                                                                                                                                                                                                                                                                                                                                                                                                       -(4.905*l2*(conj(mu6) + 2.0*conj(mu8))*(sin(q1) - 1.0*sin(q1 + q2) + q2*cos(q1 + q2)))/q2^2];

K=[0.68,0;0,0.7];
D=[0.0029,0;0,0.003];
q_dotdot=(eye(2)/M)*(torque-K*[q1;q2]-D*[qdot1;qdot2]-C_q-G);
